simulink model "mpcprueba23"  (R2025a)
settings: Solver=FixedStepAuto  StartTime=0.0  StopTime=inf  FixedStep=0.001  RelTol=1e-3  EnableMultiTasking=on
libraries: px4Sensorslib x1, px4Peripheralslib x1
settings Model: SimulationMode=external  PacingRate=0.790000  ExtModeTrigDuration=10  Creator=The MathWorks, Inc.  LastModifiedBy=aero
settings SolverCC: AlgebraicLoopSolver=TrustRegion  PositivePriorityOrder=on  AutoInsertRateTranBlk=on  MaxZcPerStep=1.0
settings OptimizationCC: EnhancedBackFolding=on  PassReuseOutputArgsAs=Individual arguments  MaxStackSize=64  OptimizeBlockOrder=speed  DifferentSizesBufferReuse=on  OptimizationCustomize=off  EfficientTunableParamExpr=on
settings DebuggingCC: ParameterPrecisionLossMsg=none  ParameterTunabilityLossMsg=error  UnconnectedInputMsg=warning  UnconnectedOutputMsg=warning  UnconnectedLineMsg=warning  SubsystemReferenceDiagnosticForUnitTest=warning  ArithmeticOperatorsInVariantConditions=warning
settings HardwareCC: ProdBitPerPointer=32.0  ProdBitPerSizeT=32.0  ProdBitPerPtrDiffT=32.0  ProdLargestAtomicInteger=Long  ProdLargestAtomicFloat=Double  ProdWordSize=32.0  ProdLongLongMode=on  ProdHWDeviceType=ARM Compatible->ARM Cortex
settings ModelReferenceCC: EnableRefExpFcnMdlSchedulingChecks=on
settings SFSimCC: MATLABDynamicMemAlloc=off  SimTargetLang=C++  SimDLTargetLibrary=mkl-dnn
settings RTWCC: SystemTargetFile=ert.tlc  HardwareBoard=PX4 Pixhawk 6c  TLCOptions="-aInlineSetEventsForThisBaseRateFcn=TLC_FALSE -aSuppressMultiTaskScheduler=TLC_FALSE  -aRateBasedStepFcn=0"  TemplateMakefile=ert_default_tmf  GenerateReport=on  Toolchain=GNU Tools for PX4 Autopilots  BuildConfiguration=Faster Runs  IncludeHyperlinkInReport=on  LaunchReport=on  TargetLang=C++  GenerateTraceInfo=on  GenerateTraceReport=on  GenerateTraceReportSl=on  GenerateTraceReportSf=on  GenerateTraceReportEml=on  GPUComputeCapability=3.5  DLArmComputeVersion=19.05  Description=Embedded Coder
settings CodeAppCC: ForceParamTrailComments=on  IgnoreCustomStorageClasses=off  OperatorAnnotations=on  SimulinkDataObjDesc=on  SFDataObjDesc=on  InsertBlockDesc=on
settings ERTTargetCC: ExtModeTransport=3.0  ExtModeStaticAllocSize=1024.0  InlinedParameterPlacement=Hierarchical

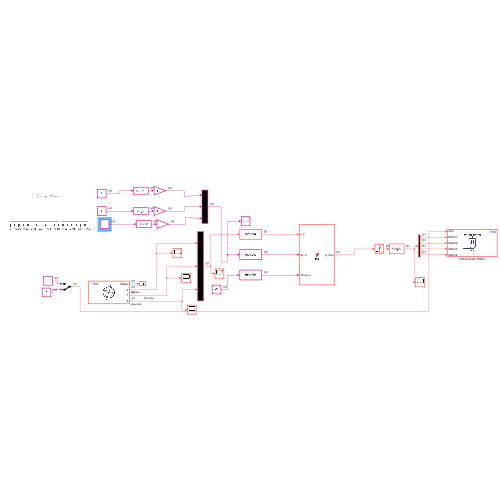
[thumbnail: Simulink's stored preview of the top-level diagram]
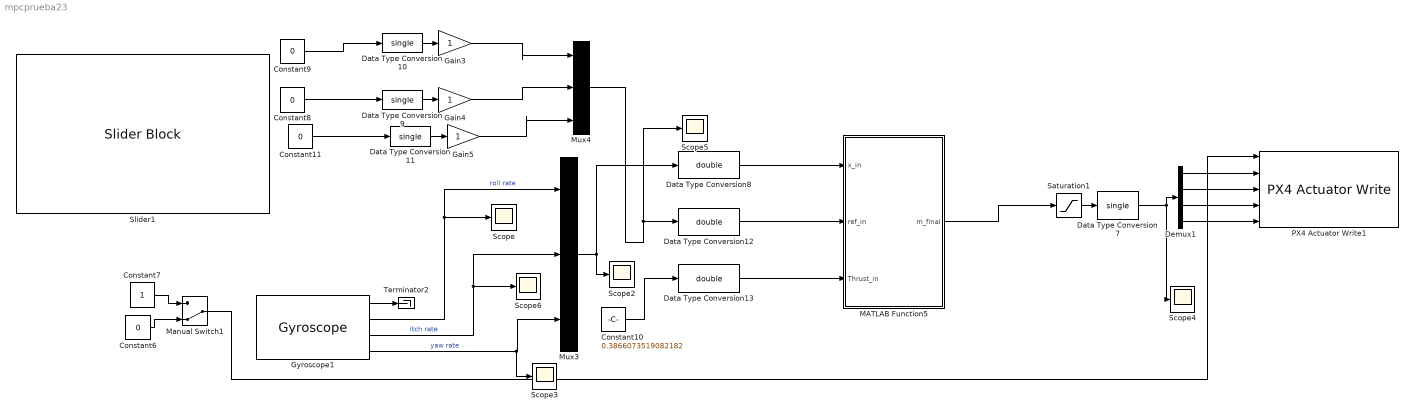
== system mpcprueba23 ==
  Constant10 : Constant  Value=0.3866073519082182
  Constant11 : Constant  Value=0
  Constant6 : Constant  Value=0  OutDataTypeStr=boolean
  Constant7 : Constant  OutDataTypeStr=boolean
  Constant8 : Constant  Value=0
  Constant9 : Constant  Value=0
  Data Type Conversion{7,9..11} (4 alike) : DataTypeConversion  OutDataTypeStr=single  SaturateOnIntegerOverflow=off  RndMeth=Floor
  Data Type Conversion12 : DataTypeConversion  OutDataTypeStr=double  SaturateOnIntegerOverflow=off  RndMeth=Floor  LockScale=on
  Data Type Conversion13 : DataTypeConversion  OutDataTypeStr=double  SaturateOnIntegerOverflow=off  RndMeth=Floor  LockScale=on
  Data Type Conversion8 : DataTypeConversion  OutDataTypeStr=double  SaturateOnIntegerOverflow=off  RndMeth=Floor  LockScale=on
  Demux1 : Demux
  Gain3 : Gain
  Gain4 : Gain
  Gain5 : Gain
  Gyroscope1 : px4Sensorslib/Gyroscope  uorbTimeStamp=off  BlockingMode=off  BlockTimeout=1e-3  sampleTime=0.001
  MATLAB Function5 : MATLAB Function  TreatAsAtomicUnit=on
  Manual Switch1 : ManualSwitch  CurrentSetting=0
  Mux3 : Mux  Inputs=3
  Mux4 : Mux  Inputs=3
  PX4 Actuator Write1 : px4Peripheralslib/PX4 Actuator Write  Motor1Enable=on  Motor2Enable=on  Motor3Enable=on  Motor4Enable=on  Motor5Enable=off  Motor6Enable=off  Motor7Enable=off  Motor8Enable=off  Motor9Enable=off  Motor10Enable=off  Motor11Enable=off  Motor12Enable=off  IsMotorArray=off  Servo1Enable=off  Servo2Enable=off  Servo3Enable=off  Servo4Enable=off  Servo5Enable=off  Servo6Enable=off  Servo7Enable=off  Servo8Enable=off  IsServoArray=off
  Saturation1 : Saturate  UpperLimit=1  LowerLimit=0
  Scope{,2..6} (6 alike) : Scope
      Scope settings: ActiveDisplayYMinimum=-0.048647073097527027  ActiveDisplayYMaximum=0.043675837107002735
      Scope2 settings: ActiveDisplayYMinimum=-0.62053689360618591  ActiveDisplayYMaximum=0.55083355307579041
      Scope3 settings: ActiveDisplayYMinimum=-1  ActiveDisplayYMaximum=1  DataLoggingVariableName=ScopeData3
      Scope4 settings: ActiveDisplayYMinimum=0.057510972242240666  ActiveDisplayYMaximum=0.55490137269269046  DataLoggingVariableName=ScopeData4
      Scope5 settings: ActiveDisplayYMinimum=-1  ActiveDisplayYMaximum=1  DataLoggingVariableName=ScopeData5
      Scope6 settings: ActiveDisplayYMinimum=-1  ActiveDisplayYMaximum=1  DataLoggingVariableName=ScopeData6
  Slider1 : SliderBlock  ScaleMax=0.6
  Terminator2 : Terminator
  wires:
  Constant11/1 -> Data Type Conversion11/1
  Constant8/1 -> Data Type Conversion9/1
  Gain4/1 -> Mux4/2
  Data Type Conversion7/1 -> Demux1/1, Scope4/1
  Data Type Conversion9/1 -> Gain4/1
  Demux1/1 -> PX4 Actuator Write1/2
  Saturation1/1 -> Data Type Conversion7/1
  Mux4/1 -> Scope5/1, Data Type Conversion12/1
  Demux1/4 -> PX4 Actuator Write1/5
  Gyroscope1/4 -> Scope3/1, Mux3/3  "yaw rate"
  Mux3/1 -> Scope2/1, Data Type Conversion8/1
  Gyroscope1/1 -> Terminator2/1
  Data Type Conversion11/1 -> Gain5/1
  Manual Switch1/1 -> PX4 Actuator Write1/1
  Data Type Conversion8/1 -> MATLAB Function5/1(x_in)
  Data Type Conversion10/1 -> Gain3/1
  Constant10/1 -> Data Type Conversion13/1
  Gain3/1 -> Mux4/1
  Gyroscope1/2 -> Scope/1, Mux3/1  "roll rate"
  Constant6/1 -> Manual Switch1/2
  Constant9/1 -> Data Type Conversion10/1
  Gain5/1 -> Mux4/3
  Gyroscope1/3 -> Mux3/2, Scope6/1  "itch rate"
  Demux1/2 -> PX4 Actuator Write1/3
  Constant7/1 -> Manual Switch1/1
  MATLAB Function5/1(m_final) -> Saturation1/1
  Demux1/3 -> PX4 Actuator Write1/4
  Data Type Conversion13/1 -> MATLAB Function5/3(Thrust_in)
  Data Type Conversion12/1 -> MATLAB Function5/2(ref_in)

== matlab function mpcprueba23/MATLAB Function5 ==
  data: x_in input; m_final output; ref_in input; Thrust_in input
function m_final = fcn(x_in, ref_in, Thrust_in)
%#codegen

% --- CONFIGURACIÓN ESTÁTICA ---
persistent A B Phi F_f H M options lb ub Q_big
    
if isempty(A)
    % 1. Matrices del sistema
    A = [ 0.9347,  0.0728,  0.6931;
          0.0043,  0.9492,  0.1273;
         -0.0283, -0.0333,  0.7369];
    B = [ 0.0094, -0.0779, -0.2379;
         -0.0359,  0.1212, -0.0441;
          0.1047,  0.0299,  0.0955];
        
    % Pre-dimensionado total (N=6, nx=3, nu=3 -> 18)
    F_mat = zeros(18, 3);
    Phi_mat = zeros(18, 18);
    Q_big_mat = zeros(18, 18);
    R_big_mat = zeros(18, 18);
    
    Q_inst = eye(3) * 1; 
    R_inst = eye(3) * 2; 
        
    % Llenado de matrices con índices fijos para el compilador
    for i = 1:6
        row = (i-1)*3 + (1:3); % Esto es aceptado por Coder
        F_mat(row, :) = A^i;
        Q_big_mat(row, row) = Q_inst;
        R_big_mat(row, row) = R_inst;
        
        for j = 1:i
            col = (j-1)*3 + (1:3);
            Phi_mat(row, col) = A^(i-j) * B;
        end
    end
        
    H = 2 * (Phi_mat' * Q_big_mat * Phi_mat + R_big_mat);
    F_f = 2 * Phi_mat' * Q_big_mat * F_mat;
    Phi = Phi_mat; 
    Q_big = Q_big_mat;
        
    M = [ -1,  1,  1, -1; 
           1, -1,  1, -1; 
          -1, -1,  1,  1; 
           1,  1,  1,  1 ];
           
    options = optimoptions('quadprog', 'Algorithm', 'active-set', 'Display', 'off');
    
    % Definición directa de límites
    lb = -2 * ones(18, 1); 
    ub =  2 * ones(18, 1);
end

% --- PROCESAMIENTO ---
x = double(x_in(:));
ref_vec = double(ref_in(:));
Thrust_Cmd = double(Thrust_in);

% --- LÓGICA MPC ---
U0 = zeros(18, 1); 
Ref_seq = repmat(ref_vec, 6, 1);
f = F_f * x - (2 * Phi' * Q_big * Ref_seq);
    
[U_sol, ~, exitflag] = quadprog(H, f, [], [], [], [], lb, ub, U0, options);
    
u = zeros(3,1);
if exitflag > 0
    u = U_sol(1:3);
end
    
% Mezcla final
u_total = [u(1); u(2); u(3); Thrust_Cmd * 4]; 
m_calc = M \ u_total; 
m_final = max(min(m_calc, 1.0), 0.0);

end
